simulink model "CVS_code"  (R2025b)
settings: Solver=ode1  StartTime=0.0  StopTime=100  FixedStep=1e-3  RelTol=1e-3
settings Model: SimulationMode=accelerator  Creator=ehd  LastModifiedBy=ehd

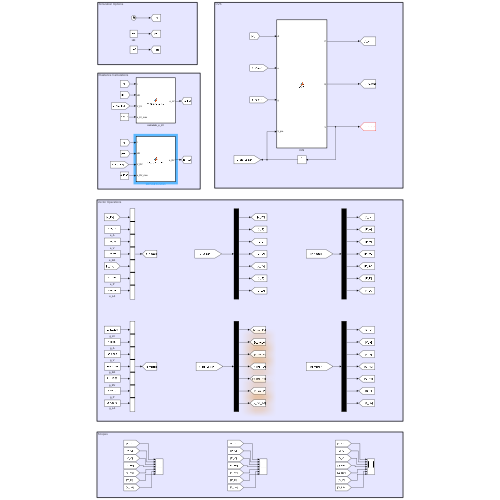
[thumbnail: Simulink's stored preview of the top-level diagram]
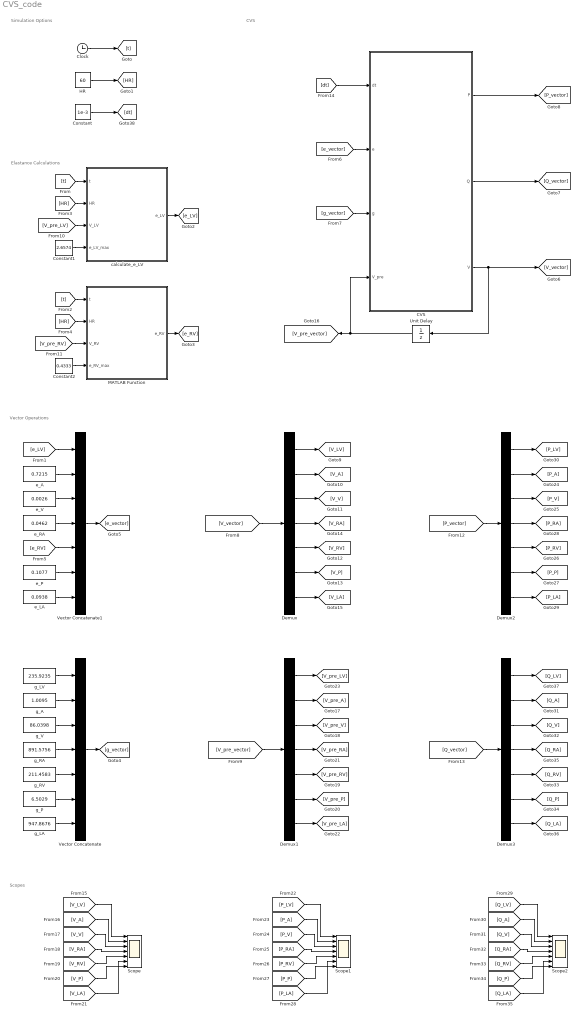
== system CVS_code ==
  note: Scopes
  note: Simulation Options
  note: CVS
  note: Elastance Calculations
  note: Vector Operations
  CVS : MATLAB Function  TreatAsAtomicUnit=on
  Clock : Clock
  Constant : Constant  Value=1e-3  OutDataTypeStr=double
  Constant1 : Constant  Value=2.6574
  Constant2 : Constant  Value=0.4333
  Demux{,1..3} (4 alike) : Demux  Outputs=7
  HR : Constant  Value=60
  MATLAB Function : MATLAB Function  TreatAsAtomicUnit=on
  Scope : Scope  NumInputPorts=7
      settings: ActiveDisplayYMinimum=-439.48350684520477  ActiveDisplayYMaximum=499.41737470393508
  Scope1 : Scope  NumInputPorts=7
      settings: ActiveDisplayYMinimum=-13.755387466131941  ActiveDisplayYMaximum=138.19772034494406
  Scope2 : Scope  NumInputPorts=7
      settings: ActiveDisplayYMinimum=4115.4174557174438  ActiveDisplayYMaximum=4723.4324390890561  DataLoggingVariableName=ScopeData2
  Unit Delay : UnitDelay  InitialCondition=[0; 0; 5000; 0; 0; 0; 0]  SampleTime=-1  HasFrameUpgradeWarning=on
  Vector Concatenate : Concatenate  NumInputs=7
  Vector Concatenate1 : Concatenate  NumInputs=7
  calculate_e_LV : MATLAB Function  TreatAsAtomicUnit=on
  e_A : Constant  Value=0.7215
  e_LA : Constant  Value=0.0938
  e_P : Constant  Value=0.1077
  e_RA : Constant  Value=0.0462
  e_V : Constant  Value=0.0026
  g_A : Constant  Value=1.0095
  g_LA : Constant  Value=947.8676
  g_LV : Constant  Value=235.9235
  g_P : Constant  Value=6.5029
  g_RA : Constant  Value=891.5756
  g_RV : Constant  Value=211.4583
  g_V : Constant  Value=86.0398
  wires:
  Clock/1 -> [t]
  [t] -> calculate_e_LV/1(t)
  [t] -> MATLAB Function/1(t)
  HR/1 -> [HR]
  [HR] -> calculate_e_LV/2(HR)
  [HR] -> MATLAB Function/2(HR)
  calculate_e_LV/1(e_LV) -> [e_LV]
  MATLAB Function/1(e_RV) -> [e_RV]
  g_LV/1 -> Vector Concatenate/1
  g_A/1 -> Vector Concatenate/2
  g_V/1 -> Vector Concatenate/3
  g_RA/1 -> Vector Concatenate/4
  g_RV/1 -> Vector Concatenate/5
  g_P/1 -> Vector Concatenate/6
  g_LA/1 -> Vector Concatenate/7
  Vector Concatenate/1 -> [g_vector]
  Vector Concatenate1/1 -> [e_vector]
  e_LA/1 -> Vector Concatenate1/7
  e_P/1 -> Vector Concatenate1/6
  [e_RV] -> Vector Concatenate1/5
  e_RA/1 -> Vector Concatenate1/4
  e_V/1 -> Vector Concatenate1/3
  e_A/1 -> Vector Concatenate1/2
  [e_LV] -> Vector Concatenate1/1
  [e_vector] -> CVS/2(e)
  [g_vector] -> CVS/3(g)
  CVS/3(V) -> Unit Delay/1, [V_vector]
  Unit Delay/1 -> [V_pre_vector], CVS/4(V_pre)
  CVS/2(Q) -> [Q_vector]
  CVS/1(P) -> [P_vector]
  [V_vector] -> Demux/1
  Demux/1 -> [V_LV]
  Demux/2 -> [V_A]
  Demux/3 -> [V_V]
  Demux/4 -> [V_RA]
  Demux/5 -> [V_RV]
  Demux/6 -> [V_P]
  Demux/7 -> [V_LA]
  [V_pre_LV] -> calculate_e_LV/3(V_LV)
  [V_pre_RV] -> MATLAB Function/3(V_RV)
  Constant1/1 -> calculate_e_LV/4(e_LV_max)
  Constant2/1 -> MATLAB Function/4(e_RV_max)
  [V_pre_vector] -> Demux1/1
  Demux1/1 -> [V_pre_LV]
  Demux1/2 -> [V_pre_A]
  Demux1/3 -> [V_pre_V]
  Demux1/4 -> [V_pre_RA]
  Demux1/5 -> [V_pre_RV]
  Demux1/6 -> [V_pre_P]
  Demux1/7 -> [V_pre_LA]
  Demux2/7 -> [P_LA]
  Demux2/6 -> [P_P]
  Demux2/5 -> [P_RV]
  Demux2/4 -> [P_RA]
  Demux2/3 -> [P_V]
  Demux2/2 -> [P_A]
  Demux2/1 -> [P_LV]
  [P_vector] -> Demux2/1
  [Q_vector] -> Demux3/1
  Demux3/1 -> [Q_LV]
  Demux3/2 -> [Q_A]
  Demux3/3 -> [Q_V]
  Demux3/4 -> [Q_RA]
  Demux3/5 -> [Q_RV]
  Demux3/6 -> [Q_P]
  Demux3/7 -> [Q_LA]
  Constant/1 -> [dt]
  [dt] -> CVS/1(dt)
  [V_LV] -> Scope/1
  [V_A] -> Scope/2
  [V_V] -> Scope/3
  [V_RA] -> Scope/4
  [V_RV] -> Scope/5
  [V_P] -> Scope/7
  [V_LA] -> Scope/6
  [P_LA] -> Scope1/6
  [P_P] -> Scope1/7
  [P_RV] -> Scope1/5
  [P_RA] -> Scope1/4
  [P_V] -> Scope1/3
  [P_A] -> Scope1/2
  [P_LV] -> Scope1/1
  [Q_LV] -> Scope2/1
  [Q_A] -> Scope2/2
  [Q_V] -> Scope2/3
  [Q_RA] -> Scope2/4
  [Q_RV] -> Scope2/5
  [Q_P] -> Scope2/7
  [Q_LA] -> Scope2/6

== matlab function CVS_code/MATLAB Function ==
  data: t input; HR input; e_RV output; V_RV input; e_RV_max input
function e_RV = calculate_e_RV(t, HR, V_RV, e_RV_max)
    k_0 = (-0.0042 * HR * HR - 0.0417 * HR + 257.5) / 1000.0;
    k_1 = (0.0158 * HR * HR - 5.0417 * HR + 445.5) / 1000.0;

    a_3 = 0.03752;
    b_3 = 0.03776;
    % d_3 = 0.2107;
    c_erv = 150.1;
    e_min_RV = a_3 * (exp(b_3 * (V_RV - c_erv)) + 1.0);

    HR = 60;
    freq   = HR / 60.0;
    tbeat = mod(t, 1.0 / freq);
    th    = 1.0 / freq;
    tce   = k_0 + k_1 * th;

    a_phi = 0.9;
    b_phi = 0.25;

    if tbeat >= 0.0 && tbeat < tce
        phi = a_phi * sin((pi * tbeat) / tce) - b_phi * sin((2.0 * pi * tbeat) / tce);
    else 
        phi = 0.0;
    end

    e_RV = e_min_RV * (1.0 - phi) + e_RV_max * phi;
end

== matlab function CVS_code/calculate_e_LV ==
  data: t input; HR input; e_LV output; V_LV input; e_LV_max input
function e_LV = calculate_e_LV(t, HR, V_LV, e_LV_max)
    a_lv  = 0.4641;
    d_lv  = 0.1235;
    b_lv  = 0.018;
    c_lv  = 145.0;

    e_LV_min = a_lv * (exp(b_lv * (V_LV - c_lv)) - 1.0) + d_lv;

    freq   = HR / 60.0;
    tbeat = mod(t, 1.0 / freq);
    tes   = 0.35 / freq;
    tn    = tbeat / tes;

    c1    = 461.4567;
    c2    = 126.2886;
    c3    = 333.3319;
    c4    = 0.3789;
    beta  = 1.9;
    gamma = 37.0;
    delta = 38.9;
    alpha = 1.5;

    d  = c2 + c3 * tn^(beta) + c4 * tn^(gamma) + tn^(delta);
    en = (c1 * tn^(alpha)) / d;
    
    e_LV = (e_LV_max - e_LV_min) * en + e_LV_min;
end

== matlab function CVS_code/CVS ==
  data: dt input; P output; e input; g input; V_pre input; Q output; V output
function [P, Q, V] = CVS(dt, e, g, V_pre)
    P = zeros(7, 1);
    Q = zeros(7, 1);
    V = zeros(7, 1);
    
    % Elastances
    e_LV = e(1);
    e_A  = e(2);
    e_V  = e(3);
    e_RA = e(4);
    e_RV = e(5);
    e_P  = e(6);
    e_LA = e(7);

    % Admittances
    g_LV = g(1);
    g_A  = g(2);
    g_V  = g(3);
    g_RA = g(4);
    g_RV = g(5);
    g_P  = g(6);
    g_LA = g(7);
    
    % Previous Volumes
    V_pre_LV = V_pre(1);
    V_pre_A  = V_pre(2);
    V_pre_V  = V_pre(3);
    V_pre_RA = V_pre(4);
    V_pre_RV = V_pre(5);
    V_pre_P  = V_pre(6);
    V_pre_LA = V_pre(7);
    
    % calculate elastances
    % e_LV = calculate_e_LV(t, V_pre_LV, e_LV_max);
    % e_RV = calculate_e_RV(t, V_pre_RV, e_RV_max);

    % calculate pressures
    P(1) = e_LV * V_pre_LV;
    P(2) = e_A  * V_pre_A;
    P(3) = e_V  * V_pre_V;
    P(4) = e_RA * V_pre_RA;
    P(5) = e_RV * V_pre_RV;
    P(6) = e_P  * V_pre_P;
    P(7) = e_LA * V_pre_LA;

    % assign pressures
    P_LV = P(1);
    P_A  = P(2);
    P_V  = P(3);
    P_RA = P(4);
    P_RV = P(5);
    P_P  = P(6);
    P_LA = P(7);

    % calculate flows
    Q(1) = g_LV * max(0, (P_LV - P_A));
    Q(2) = g_A  * (P_A  - P_V);
    Q(3) = g_V  * (P_V  - P_RA);
    Q(4) = g_RA * max(0, (P_RA - P_RV));
    Q(5) = g_RV * max(0, (P_RV - P_P));
    Q(6) = g_P  * (P_P  - P_LA);
    Q(7) = g_LA * max(0, (P_LA - P_LV));

    % assign flows
    Q_LV = Q(1);
    Q_A  = Q(2);
    Q_V  = Q(3);
    Q_RA = Q(4);
    Q_RV = Q(5);
    Q_P  = Q(6);
    Q_LA = Q(7);

    % calculate volume changes
    q_LV = Q_LA - Q_LV;
    q_A  = Q_LV - Q_A;
    q_V  = Q_A  - Q_V;
    q_RA = Q_V  - Q_RA;
    q_RV = Q_RA - Q_RV;
    q_P  = Q_RV - Q_P;
    q_LA = Q_P  - Q_LA;

    % update volumes
    V(1) = V_pre_LV + q_LV * dt;
    V(2) = V_pre_A  + q_A  * dt;
    V(3) = V_pre_V  + q_V  * dt;
    V(4) = V_pre_RA + q_RA * dt;
    V(5) = V_pre_RV + q_RV * dt;
    V(6) = V_pre_P  + q_P  * dt;
    V(7) = V_pre_LA + q_LA * dt;
end
